simulink model "Push_Button_EdgeDetection"  (R2015b)
settings: Solver=FixedStepDiscrete  StartTime=0.0  StopTime=1  RelTol=1e-3
libraries: simulink x14, stm32f4lib x5, dspswit3 x1
settings Model: Creator=ronak  LastModifiedBy=ronak
settings OptimizationCC: OptimizeModelRefInitCode=on  LifeSpan=1  MaxStackSize=64
settings HardwareCC: ProdBitPerPointer=32  ProdLargestAtomicInteger=Long  ProdLargestAtomicFloat=Double  ProdWordSize=32  ProdHWDeviceType=ARM Compatible->ARM Cortex
settings RTWCC: SystemTargetFile=ert.tlc  TemplateMakefile=ert_default_tmf  Description=Embedded Coder  GenerateReport=on  Toolchain=GNU Tools for ARM Embedded Processors  IncludeHyperlinkInReport=on  LaunchReport=on  GenerateTraceInfo=on  GenerateTraceReport=on  GenerateTraceReportSl=on  GenerateTraceReportSf=on  GenerateTraceReportEml=on  GenerateWebview=on
settings CodeAppCC: IgnoreCustomStorageClasses=off

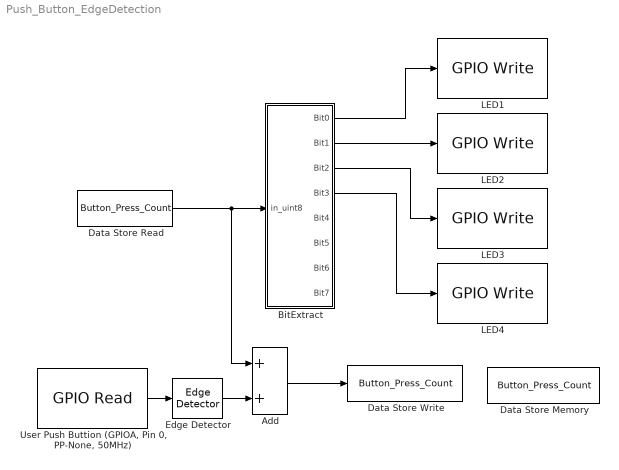
== system Push_Button_EdgeDetection ==
  Add : Sum
  BitExtract : Subsystem
  Data Store Memory : DataStoreMemory  DataStoreName=Button_Press_Count  ReadBeforeWriteMsg=warning  WriteAfterWriteMsg=warning  WriteAfterReadMsg=warning  OutDataTypeStr=uint8
      settings: RTWStateStorageClass=ExportedGlobal
  Data Store Read : DataStoreRead  DataStoreName=Button_Press_Count
  Data Store Write : DataStoreWrite  DataStoreName=Button_Press_Count
  Edge Detector : dspswit3/Edge Detector  InputProcessing=Columns as channels (frame based)
  LED1 : stm32f4lib/GPIO Write  gpio_name=GPIOD  pin_number=12  pupd_reg=0  otype_reg=0  ospeed_reg=0  gpio_init_out=off  toggle_pin=off
  LED2 : stm32f4lib/GPIO Write  gpio_name=GPIOD  pin_number=13  pupd_reg=0  otype_reg=0  ospeed_reg=0  gpio_init_out=off  toggle_pin=off
  LED3 : stm32f4lib/GPIO Write  gpio_name=GPIOD  pin_number=14  pupd_reg=0  otype_reg=0  ospeed_reg=0  gpio_init_out=off  toggle_pin=off
  LED4 : stm32f4lib/GPIO Write  gpio_name=GPIOD  pin_number=15  pupd_reg=0  otype_reg=0  ospeed_reg=0  gpio_init_out=off  toggle_pin=off
  "User Push Buttion (GPIOA, Pin 0, PP-None, 50MHz)" : stm32f4lib/GPIO Read  gpio_name=GPIOA  pin_number=0  sample_time=0.1  pupd_reg=0  otype_reg=0  ospeed_reg=0
  wires:
  Add/1 -> Data Store Write/1
  Data Store Read/1 -> Add/1, BitExtract/1(in_uint8)
  "User Push Buttion (GPIOA, Pin 0, PP-None, 50MHz)"/1 -> Edge Detector/1
  Edge Detector/1 -> Add/2
  BitExtract/1(Bit0) -> LED1/1
  BitExtract/2(Bit1) -> LED2/1
  BitExtract/3(Bit2) -> LED3/1
  BitExtract/4(Bit3) -> LED4/1

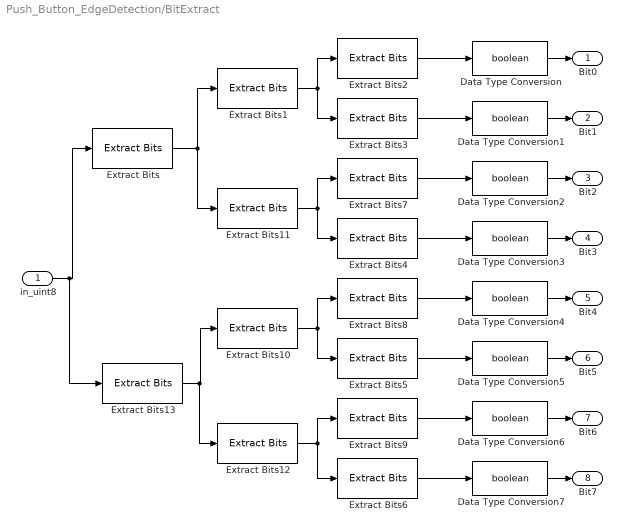
== system Push_Button_EdgeDetection/BitExtract ==
  in_uint8 : Inport
  Data Type Conversion{,1..7} (8 alike) : DataTypeConversion  OutDataTypeStr=boolean
  Extract Bits{,1..2,7..10} (7 alike) : simulink/Logic and Bit Operations/Extract Bits  bitsToExtract=Lower half  numBits=8  bitIdxRange=[0 7]  outScalingMode=Treat bit field as an integer
  Extract Bits{3..6,11..13} (7 alike) : simulink/Logic and Bit Operations/Extract Bits  bitsToExtract=Upper half  numBits=8  bitIdxRange=[0 7]  outScalingMode=Treat bit field as an integer
  Bit0 : Outport
  Bit1 : Outport  Port=2
  Bit2 : Outport  Port=3
  Bit3 : Outport  Port=4
  Bit4 : Outport  Port=5
  Bit5 : Outport  Port=6
  Bit6 : Outport  Port=7
  Bit7 : Outport  Port=8
  wires:
  Extract Bits2/1 -> Data Type Conversion/1
  Extract Bits1/1 -> Extract Bits2/1, Extract Bits3/1
  Extract Bits/1 -> Extract Bits1/1, Extract Bits11/1
  in_uint8/1 -> Extract Bits13/1, Extract Bits/1
  Extract Bits3/1 -> Data Type Conversion1/1
  Extract Bits5/1 -> Data Type Conversion5/1
  Extract Bits6/1 -> Data Type Conversion7/1
  Extract Bits7/1 -> Data Type Conversion2/1
  Extract Bits4/1 -> Data Type Conversion3/1
  Extract Bits8/1 -> Data Type Conversion4/1
  Extract Bits9/1 -> Data Type Conversion6/1
  Extract Bits12/1 -> Extract Bits9/1, Extract Bits6/1
  Extract Bits10/1 -> Extract Bits8/1, Extract Bits5/1
  Extract Bits11/1 -> Extract Bits4/1, Extract Bits7/1
  Extract Bits13/1 -> Extract Bits12/1, Extract Bits10/1
  Data Type Conversion/1 -> Bit0/1
  Data Type Conversion1/1 -> Bit1/1
  Data Type Conversion2/1 -> Bit2/1
  Data Type Conversion3/1 -> Bit3/1
  Data Type Conversion4/1 -> Bit4/1
  Data Type Conversion5/1 -> Bit5/1
  Data Type Conversion6/1 -> Bit6/1
  Data Type Conversion7/1 -> Bit7/1
